simulink model "PV_MPPT"  (R2024a)
settings: Solver=ode23tb  StartTime=0.0  StopTime=10  RelTol=1e-4
libraries: spsSeriesRLCBranchLib x13, spsIGBTDiodeLib x6, spsGroundLib x3, spsSawtoothGeneratorLib x3, spsCurrentMeasurementLib x3, spsThreePhaseVIMeasurementLib x2, spsMeanLib x2, spsVoltageMeasurementLib x2, spspowerguiLib x1, simulink x1, spsDiodeLib x1, spsIGBTLib x1
settings Model: Creator=91889  LastModifiedBy=91889

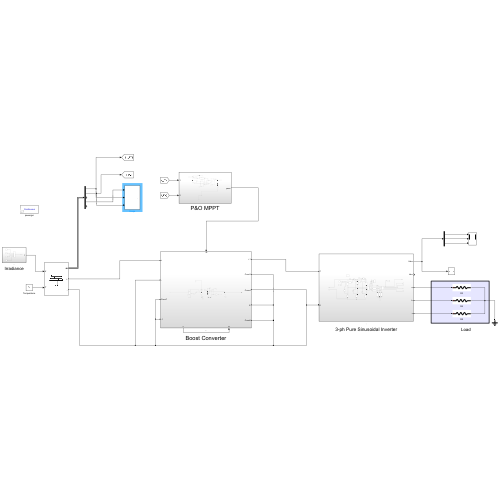
[thumbnail: Simulink's stored preview of the top-level diagram]
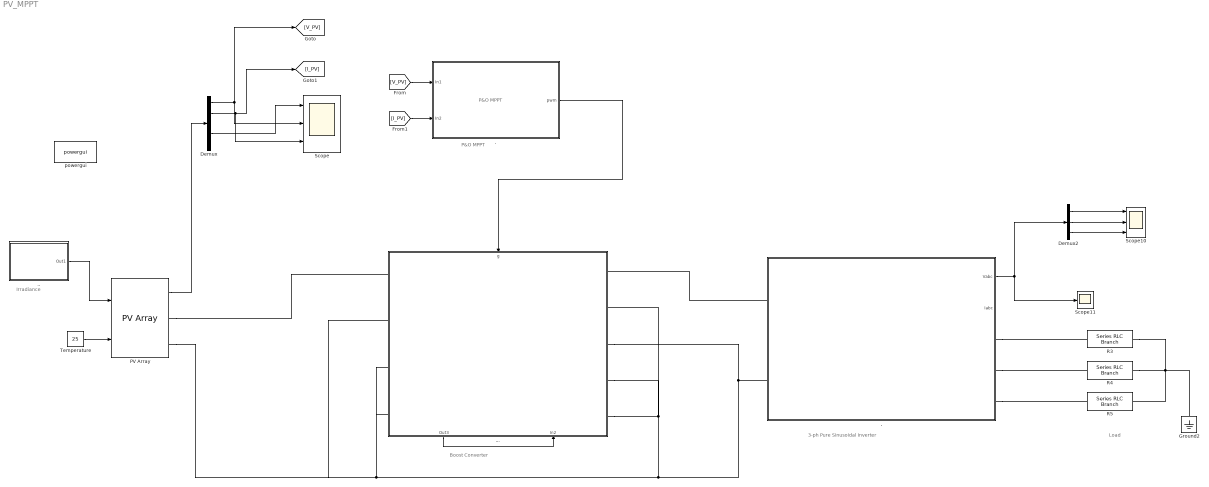
== system PV_MPPT ==
  note: Load
  note: 3-ph Pure Sinusoidal Inverter
  note: Boost Converter
  note: Irradiance
  note: P&O MPPT
  note: P&O MPPT
  , : Subsystem
  . : Subsystem
  .. : Subsystem
  ... : Subsystem
      settings: PortSchema="{\"entries\":[{\"content\":{\"sides\":[{\"content\":{\"connectorIds\":[\"LConn1\",\"LConn2\",\"LConn3\",\"LConn4\"]},\"type\":\"ConnectorPlacement.EquallySpacedRectSide\",\"uuid\":\"853841bf-2c6c-476b-8930-0dad7cd27bd4\"},{\"content\":{\"connectorIds\":[\"RConn1\",\"RConn2\",\"RConn3\",\"RConn4\",\"RConn5\"],\"side\":\"RIGHT\"},\"type\":\"ConnectorPlacement.EquallySpacedRectSide\",\"uuid\":\"d1ca2537-bf77-4a41-a82f-700dc7148288\"},{\"content\":{\"connectorIds\":[\"In1\"],\"side\":\"TOP\"},\"type\":\"ConnectorPlacement.EquallySpacedRectSide\",\"uuid\":\"50e3e9f4-8721-4df0-9f81-d71172613d0c\"},{\"content\":{\"connectorIds\":[\"Out1\",\"In2\"],\"side\":\"BOTTOM\"},\"type\":\"ConnectorPlacement.EquallySpacedRectSide\",\"uuid\":\"0662db4a-a60b-41ea-b11c-bd3a3f86f72a\"}]},\"type\":\"ConnectorPlacement.EquallySpacedConnector\",\"uuid\":\"eb88438f-1bf4-4f6a-82c1-55dd1ddf17b5\"}],\"packageUris\":[\"http://schema.mathworks.com/mf0/Connector/R2020b\"],\"version\":\"1.0\"}"
  Demux : Demux  Outputs=5
  Demux2 : Demux  Outputs=3
  Ground2 : spsGroundLib/Ground  LConnTagsString=a
  PV Array : spsPVArrayLib/PV Array  Npar=3  Nser=20  PlotType=array @ 1000 W/m2 & specified temperatures  S_vec="[ 1000  500  100 ]"  Temp_C_vec="[ 45 25  ]"  ModuleName=User-defined  PlotWhenSelected=off  Pm=213.15  Ncell=60  Voc=35  Isc=7.84  Vm=29  Im=7.35  beta_Voc_pc=-0.36099  alpha_Isc_pc=0.102  beta_Voc=-0.12635  alpha_Isc=0.0079968  IL=7.8812  I0=2.9282e-10  nI=0.94636  Rsh=184.8932  Rs=0.22133  RobustModel=off  RobustCellTemperature=313.3991  BAL=on  Tc=1e-6  Tfilter=5e-5
  R3 : spsSeriesRLCBranchLib/Series RLC Branch  LConnTagsString=__new0  RConnTagsString=__new0  BranchType=R  Resistance=10  Inductance=1e-3  SetiL0=off  InitialCurrent=0  Capacitance=1e-6  Setx0=off  InitialVoltage=0  Measurements=None
  R4 : spsSeriesRLCBranchLib/Series RLC Branch  LConnTagsString=__new0  RConnTagsString=__new0  BranchType=R  Resistance=10  Inductance=1e-3  SetiL0=off  InitialCurrent=0  Capacitance=1e-6  Setx0=off  InitialVoltage=0  Measurements=None
  R5 : spsSeriesRLCBranchLib/Series RLC Branch  LConnTagsString=__new0  RConnTagsString=__new0  BranchType=R  Resistance=10  Inductance=1e-3  SetiL0=off  InitialCurrent=0  Capacitance=1e-6  Setx0=off  InitialVoltage=0  Measurements=None
  Scope : Scope  NumInputPorts=3
  Scope10 : Scope  NumInputPorts=3
  Scope11 : Scope
  Temperature : Constant  Value=25
  powergui : sps_lib/powergui  Priority=1  SimulationMode=Continuous  SampleTime=50e-6  frequency=60  Iterations=50  frequencyindice=0  Pbase=100e6  ErrMax=1e-4  UnitsV=kV  UnitsW=MW  buscounter=0  FunctionMessages=off  echomessages=off  EnableUseOfTLC=off  CurrentSourceSwitches=off  DisableSnubberDevices=off  DisableRonSwitches=off  DisableVfSwitches=off  DisplayEquations=off  AutomaticDiscreteSolvers=off  SolverType=Tustin/Backward Euler (TBE)  Interpol=off  ExternalGateDelay=off  methode=off  Ts=100  x0status=blocks  SPID=on  SwTol=0  HookPort=off  NonlinearTolerance=1e-4  nMaxIteration=100  ContinueOnMaxIteration=off  RestoreLinks=warning  ResistiveCurrentMeasurement=off  Frange=[0:2:500]  Ylog=off  Xlog=on  ShowGrid=off  save=off  variable=ZData  structure=0  ZoomFFT=off  StartTime=0.0  cycles=1  DisplayStyle=1  fundamental=60  FreqAxis=off  MaxFrequency=1000  frequencyindicesteady=1  RmsSteady=1  display=off
  wires:
  Temperature/1 -> PV Array/2
  PV Array/1 -> Demux/1
  Demux/1 -> [V_PV], Scope/2
  Demux/2 -> Scope/3, [I_PV]
  Demux2/3 -> Scope10/3
  Demux2/1 -> Scope10/1
  ,/1(Vabc) -> Demux2/1, Scope11/1
  Demux2/2 -> Scope10/2
  ../1(Out1) -> PV Array/1
  [V_PV] -> ./1(In1)
  [I_PV] -> ./2(In2)
  ./1(pwm) -> .../1(g)
  .../1(Out3) -> .../2(In2)
  Demux/4 -> Scope/1
  connections:
  R3/RConn1 -- R5/RConn1 -- Ground2/LConn1 -- R4/RConn1
  ,/RConn1 -- R3/LConn1
  ,/RConn2 -- R4/LConn1
  ,/RConn3 -- R5/LConn1
  ,/LConn2 -- .../LConn2 -- PV Array/RConn2 -- .../LConn4 -- .../LConn3 -- .../RConn5 -- .../RConn4 -- .../RConn2 -- .../RConn3
  PV Array/RConn1 -- .../LConn1
  ,/LConn1 -- .../RConn1

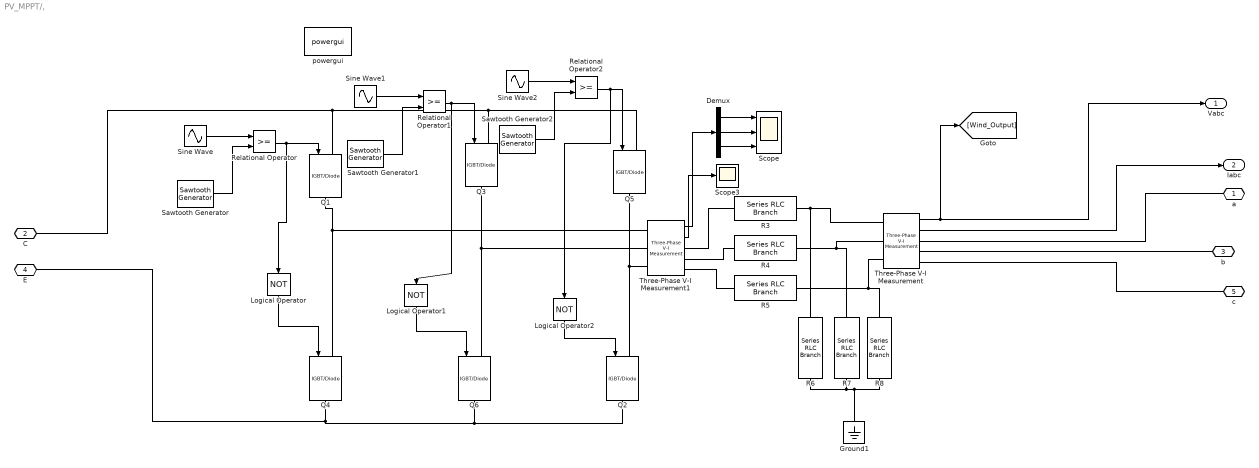
== system PV_MPPT/, ==
  Demux : Demux  Outputs=3
  Ground1 : spsGroundLib/Ground  LConnTagsString=a
  Logical Operator : Logic  Operator=NOT  AllPortsSameDT=off  OutDataTypeStr=boolean
  Logical Operator1 : Logic  Operator=NOT  AllPortsSameDT=off  OutDataTypeStr=boolean
  Logical Operator2 : Logic  Operator=NOT  AllPortsSameDT=off  OutDataTypeStr=boolean
  Q{1..6} (6 alike) : spsIGBTDiodeLib/IGBT//Diode  Ron=1e-3  Rs=1e5  Cs=inf  Measurements=off
  R3 : spsSeriesRLCBranchLib/Series RLC Branch  LConnTagsString=__new0  RConnTagsString=__new0  BranchType=L  Resistance=10  Inductance=80e-3  SetiL0=off  InitialCurrent=0  Capacitance=1e-6  Setx0=off  InitialVoltage=0  Measurements=None
  R4 : spsSeriesRLCBranchLib/Series RLC Branch  LConnTagsString=__new0  RConnTagsString=__new0  BranchType=L  Resistance=10  Inductance=80e-3  SetiL0=off  InitialCurrent=0  Capacitance=1e-6  Setx0=off  InitialVoltage=0  Measurements=None
  R5 : spsSeriesRLCBranchLib/Series RLC Branch  LConnTagsString=__new0  RConnTagsString=__new0  BranchType=L  Resistance=10  Inductance=80e-3  SetiL0=off  InitialCurrent=0  Capacitance=1e-6  Setx0=off  InitialVoltage=0  Measurements=None
  R6 : spsSeriesRLCBranchLib/Series RLC Branch  LConnTagsString=__new0  RConnTagsString=__new0  BranchType=C  Resistance=10  Inductance=80e-3  SetiL0=off  InitialCurrent=0  Capacitance=300e-6  Setx0=off  InitialVoltage=0  Measurements=None
  R7 : spsSeriesRLCBranchLib/Series RLC Branch  LConnTagsString=__new0  RConnTagsString=__new0  BranchType=C  Resistance=10  Inductance=80e-3  SetiL0=off  InitialCurrent=0  Capacitance=300e-6  Setx0=off  InitialVoltage=0  Measurements=None
  R8 : spsSeriesRLCBranchLib/Series RLC Branch  LConnTagsString=__new0  RConnTagsString=__new0  BranchType=C  Resistance=10  Inductance=80e-3  SetiL0=off  InitialCurrent=0  Capacitance=300e-6  Setx0=off  InitialVoltage=0  Measurements=None
  Relational Operator : RelationalOperator  OutDataTypeStr=boolean  InputSameDT=off
  Relational Operator1 : RelationalOperator  OutDataTypeStr=boolean  InputSameDT=off
  Relational Operator2 : RelationalOperator  OutDataTypeStr=boolean  InputSameDT=off
  Sawtooth Generator : spsSawtoothGeneratorLib/Sawtooth Generator  Freq=1000  Phase=180  Ts=0
  Sawtooth Generator1 : spsSawtoothGeneratorLib/Sawtooth Generator  Freq=1000  Phase=180  Ts=0
  Sawtooth Generator2 : spsSawtoothGeneratorLib/Sawtooth Generator  Freq=1000  Phase=180  Ts=0
  Scope : Scope  NumInputPorts=3
  Scope3 : Scope
  Sine Wave : Sin  Amplitude=0.9  Frequency=2*pi*50  SampleTime=0
  Sine Wave1 : Sin  Amplitude=0.9  Frequency=2*pi*50  Phase=120*(pi/180)  SampleTime=0
  Sine Wave2 : Sin  Amplitude=0.9  Frequency=2*pi*50  Phase=240*(pi/180)  SampleTime=0
  Three-Phase V-I Measurement : spsThreePhaseVIMeasurementLib/Three-Phase V-I Measurement  VoltageMeasurement=phase-to-phase  SetLabelV=off  LabelV=Vabc  Vpu=off  VpuLL=off  CurrentMeasurement=yes  SetLabelI=off  LabelI=Iabc  Ipu=off  Pbase=100e6  Vbase=500e3  OutputType=Complex  PhasorSimulation=off  PSBequivalent=0
  Three-Phase V-I Measurement1 : spsThreePhaseVIMeasurementLib/Three-Phase V-I Measurement  VoltageMeasurement=phase-to-phase  SetLabelV=off  LabelV=Vabc  Vpu=off  VpuLL=off  CurrentMeasurement=yes  SetLabelI=off  LabelI=Iabc  Ipu=off  Pbase=100e6  Vbase=500e3  OutputType=Complex  PhasorSimulation=off  PSBequivalent=0
  powergui : spspowerguiLib/powergui  Priority=1  SimulationMode=Continuous  SampleTime=50e-6  frequency=60  Iterations=50  frequencyindice=0  Pbase=100e6  ErrMax=1e-4  UnitsV=kV  UnitsW=MW  buscounter=0  FunctionMessages=off  echomessages=off  EnableUseOfTLC=off  CurrentSourceSwitches=off  DisableSnubberDevices=off  DisableRonSwitches=off  DisableVfSwitches=off  DisplayEquations=off  AutomaticDiscreteSolvers=off  SolverType=Tustin/Backward Euler (TBE)  Interpol=off  ExternalGateDelay=off  methode=off  Ts=100  x0status=blocks  SPID=off  SwTol=0  HookPort=off  NonlinearTolerance=1e-4  nMaxIteration=100  ContinueOnMaxIteration=off  RestoreLinks=warning  ResistiveCurrentMeasurement=off  Frange=[0:2:500]  Ylog=off  Xlog=on  ShowGrid=off  save=off  variable=ZData  structure=Vo  ZoomFFT=off  StartTime=0.0  cycles=1  DisplayStyle=1  fundamental=50  FreqAxis=on  MaxFrequency=1000  frequencyindicesteady=1  RmsSteady=1  display=off
  a : PMIOPort  Side=Right
  C : PMIOPort  Port=2  Side=Left
  b : PMIOPort  Port=3  Side=Right
  E : PMIOPort  Port=4  Side=Left
  c : PMIOPort  Port=5  Side=Right
  Vabc : Outport
  Iabc : Outport  Port=2
  wires:
  Relational Operator1/1 -> Q3/1, Logical Operator1/1
  Logical Operator/1 -> Q4/1
  Three-Phase V-I Measurement/1 -> [Wind_Output], Vabc/1
  Three-Phase V-I Measurement1/2 -> Scope3/1
  Logical Operator1/1 -> Q6/1
  Sawtooth Generator2/1 -> Relational Operator2/2
  Relational Operator2/1 -> Logical Operator2/1, Q5/1
  Logical Operator2/1 -> Q2/1
  Sawtooth Generator/1 -> Relational Operator/2
  Demux/1 -> Scope/1
  Three-Phase V-I Measurement1/1 -> Demux/1
  Relational Operator/1 -> Logical Operator/1, Q1/1
  Sawtooth Generator1/1 -> Relational Operator1/2
  Sine Wave/1 -> Relational Operator/1
  Three-Phase V-I Measurement/2 -> Iabc/1
  Sine Wave1/1 -> Relational Operator1/1
  Sine Wave2/1 -> Relational Operator2/1
  Demux/3 -> Scope/3
  Demux/2 -> Scope/2
  connections:
  R4/LConn1 -- Three-Phase V-I Measurement1/RConn2
  Q4/RConn1 -- Q6/RConn1 -- Q2/RConn1 -- E/RConn1
  Q5/LConn1 -- Q3/LConn1 -- Q1/LConn1 -- C/RConn1
  R6/LConn1 -- Three-Phase V-I Measurement/LConn1 -- R3/RConn1
  Three-Phase V-I Measurement1/LConn3 -- Q5/RConn1 -- Q2/LConn1
  Three-Phase V-I Measurement1/LConn2 -- Q3/RConn1 -- Q6/LConn1
  R7/LConn1 -- R4/RConn1 -- Three-Phase V-I Measurement/LConn2
  R5/LConn1 -- Three-Phase V-I Measurement1/RConn3
  Ground1/LConn1 -- R8/RConn1 -- R6/RConn1 -- R7/RConn1
  R8/LConn1 -- R5/RConn1 -- Three-Phase V-I Measurement/LConn3
  Three-Phase V-I Measurement/RConn3 -- c/RConn1
  Three-Phase V-I Measurement1/LConn1 -- Q1/RConn1 -- Q4/LConn1
  R3/LConn1 -- Three-Phase V-I Measurement1/RConn1
  Three-Phase V-I Measurement/RConn1 -- a/RConn1
  Three-Phase V-I Measurement/RConn2 -- b/RConn1

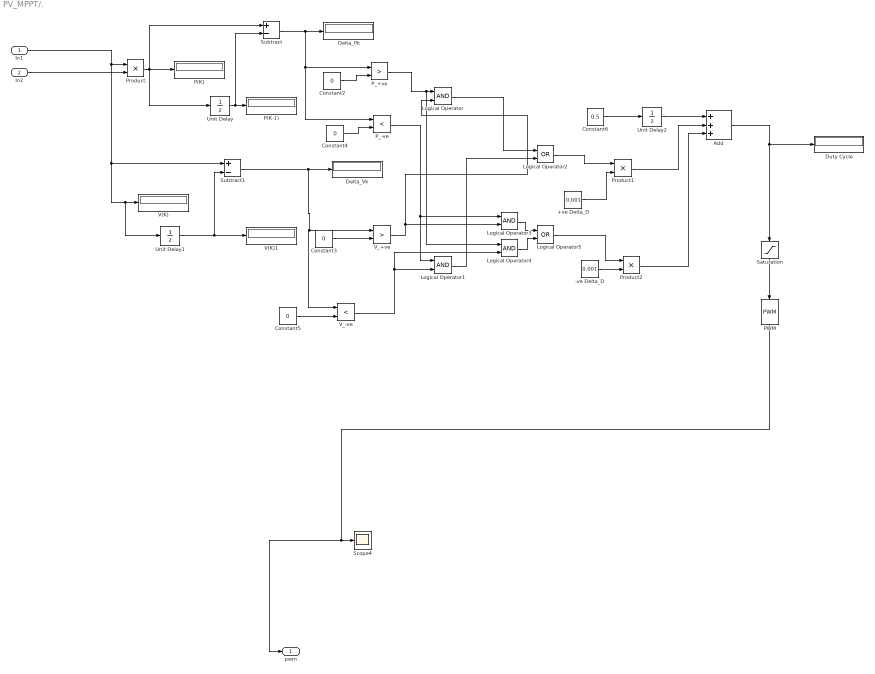
== system PV_MPPT/. ==
  In1 : Inport
  In2 : Inport  Port=2
  +ve Delta_D : Constant  Value=0.001
  -ve Delta_D : Constant  Value=0.001
  Add : Sum  Inputs=+++
  Constant{2..5} (4 alike) : Constant  Value=0
  Constant6 : Constant  Value=0.5
  Delta_Pk : Display
  Delta_Vk : Display
  Duty Cycle : Display
  Logical Operator{,1,3..4} (4 alike) : Logic  AllPortsSameDT=off  OutDataTypeStr=boolean
  Logical Operator2 : Logic  Operator=OR  AllPortsSameDT=off  OutDataTypeStr=boolean
  Logical Operator5 : Logic  Operator=OR  AllPortsSameDT=off  OutDataTypeStr=boolean
  P(K) : Display
  P(K-1) : Display
  PWM : simulink/Discontinuities/PWM  DisableCoverage=on  Period=50e-6  InitialDelay=0  DisallowZeroDutyCycle=off  RunAtFixedTimeIntervals=off  SampleTime=0.1
  P_+ve : RelationalOperator  Operator=>  OutDataTypeStr=boolean  RndMeth=Simplest  InputSameDT=off
  P_-ve : RelationalOperator  Operator=<  OutDataTypeStr=boolean  RndMeth=Simplest  InputSameDT=off
  Product : Product
  Product1 : Product
  Product2 : Product
  Saturation : Saturate  UpperLimit=0.9  LowerLimit=0.1
  Scope4 : Scope
  Subtract : Sum  Inputs=+-
  Subtract1 : Sum  Inputs=+-
  Unit Delay : UnitDelay  SampleTime=-1  HasFrameUpgradeWarning=on
  Unit Delay1 : UnitDelay  SampleTime=-1  HasFrameUpgradeWarning=on
  Unit Delay2 : UnitDelay  SampleTime=-1  HasFrameUpgradeWarning=on
  V(K) : Display
  V(K)1 : Display
  V_+ve : RelationalOperator  Operator=>  OutDataTypeStr=boolean  RndMeth=Simplest  InputSameDT=off
  V_-ve : RelationalOperator  Operator=<  OutDataTypeStr=boolean  RndMeth=Simplest  InputSameDT=off
  pwm : Outport
  wires:
  Product2/1 -> Add/3
  -ve Delta_D/1 -> Product2/2
  Product/1 -> Unit Delay/1, Subtract/1, P(K)/1
  In1/1 -> Subtract1/1, V(K)/1, Unit Delay1/1, Product/1
  +ve Delta_D/1 -> Product1/2
  V_+ve/1 -> Logical Operator/2, Logical Operator3/2
  Saturation/1 -> PWM/1
  Unit Delay1/1 -> Subtract1/2, V(K)1/1
  V_-ve/1 -> Logical Operator4/2, Logical Operator1/2
  Subtract1/1 -> V_-ve/1, V_+ve/1, Delta_Vk/1
  Logical Operator/1 -> Logical Operator2/1
  Logical Operator1/1 -> Logical Operator2/2
  Logical Operator4/1 -> Logical Operator5/2
  Add/1 -> Saturation/1, Duty Cycle/1
  Constant3/1 -> V_+ve/2
  P_+ve/1 -> Logical Operator4/1, Logical Operator/1
  Logical Operator3/1 -> Logical Operator5/1
  Constant5/1 -> V_-ve/2
  Unit Delay/1 -> Subtract/2, P(K-1)/1
  Unit Delay2/1 -> Add/1
  Subtract/1 -> Delta_Pk/1, P_-ve/1, P_+ve/1
  Constant4/1 -> P_-ve/2
  PWM/1 -> pwm/1, Scope4/1
  Constant6/1 -> Unit Delay2/1
  Product1/1 -> Add/2
  Logical Operator2/1 -> Product1/1
  Constant2/1 -> P_+ve/2
  P_-ve/1 -> Logical Operator3/1, Logical Operator1/1
  Logical Operator5/1 -> Product2/1
  In2/1 -> Product/2

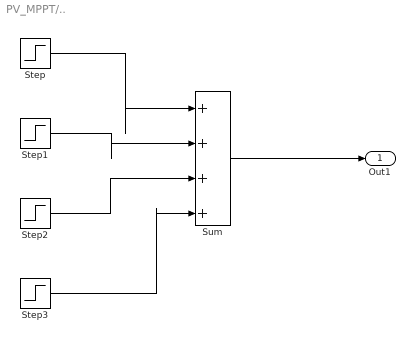
== system PV_MPPT/.. ==
  Step : Step  Time=0  Before=1200  After=1200  SampleTime=0
  Step1 : Step  Time=3  After=-300  SampleTime=0
  Step2 : Step  Time=5  After=-250  SampleTime=0
  Step3 : Step  Time=8  After=350  SampleTime=0
  Sum : Sum  Inputs=|++++
  Out1 : Outport
  wires:
  Step1/1 -> Sum/2
  Step/1 -> Sum/1
  Sum/1 -> Out1/1
  Step2/1 -> Sum/3
  Step3/1 -> Sum/4

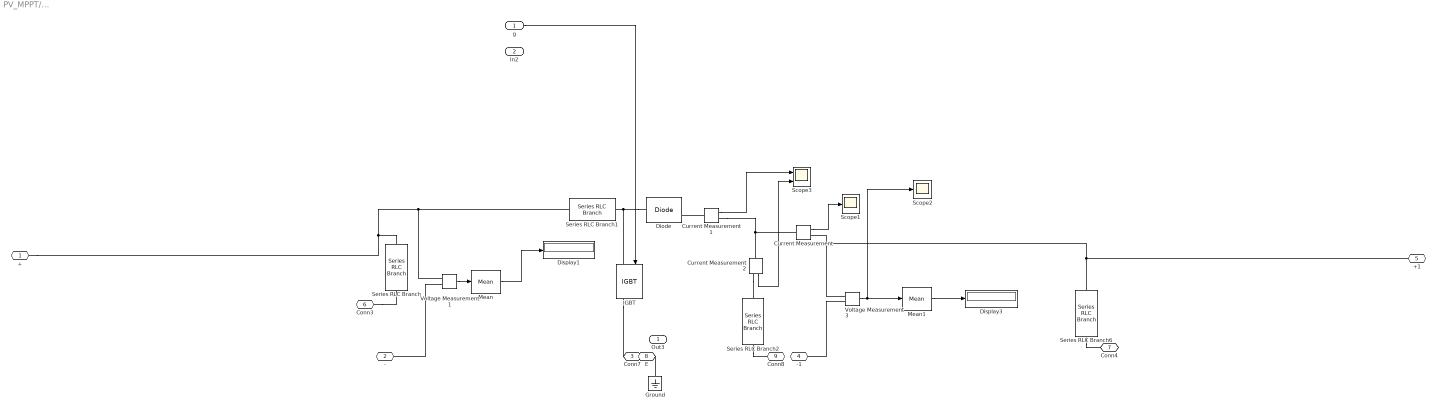
== system PV_MPPT/... ==
  g : Inport
  In2 : Inport  Port=2
  Current Measurement : spsCurrentMeasurementLib/Current Measurement  PhasorSimulation=off  OutputType=Complex  PSBequivalent=0
  Current Measurement1 : spsCurrentMeasurementLib/Current Measurement  PhasorSimulation=off  OutputType=Complex  PSBequivalent=0
  Current Measurement2 : spsCurrentMeasurementLib/Current Measurement  PhasorSimulation=off  OutputType=Complex  PSBequivalent=0
  Diode : spsDiodeLib/Diode  Ron=0.001  Lon=0  Vf=0.8  IC=0  UseSnubber=0  Rs=500  Cs=250e-9  Measurements=on
  Display1 : Display
  Display3 : Display
  Ground : spsGroundLib/Ground  LConnTagsString=a
  IGBT : spsIGBTLib/IGBT  Ron=0.001  Lon=0  Vf=1  Tf=1e-6  Tt=2e-6  IC=0  Rs=1e5  Cs=inf  Measurements=on
  Mean : spsMeanLib/Mean  Freq=60  Vinit=0  Ts=0
  Mean1 : spsMeanLib/Mean  Freq=60  Vinit=0  Ts=0
  Scope1 : Scope
  Scope2 : Scope
  Scope3 : Scope  NumInputPorts=2
  Series RLC Branch : spsSeriesRLCBranchLib/Series RLC Branch  LConnTagsString=__new0  RConnTagsString=__new0  BranchType=R  Resistance=100  Inductance=1e-3  SetiL0=off  InitialCurrent=0  Capacitance=1e-6  Setx0=off  InitialVoltage=0  Measurements=None
  Series RLC Branch1 : spsSeriesRLCBranchLib/Series RLC Branch  LConnTagsString=__new0  RConnTagsString=__new0  BranchType=L  Resistance=1  Inductance=5e-3  SetiL0=off  InitialCurrent=0  Capacitance=1e-6  Setx0=off  InitialVoltage=0  Measurements=None
  Series RLC Branch2 : spsSeriesRLCBranchLib/Series RLC Branch  LConnTagsString=__new0  RConnTagsString=__new0  BranchType=C  Resistance=1  Inductance=1e-3  SetiL0=off  InitialCurrent=0  Capacitance=1000e-6  Setx0=off  InitialVoltage=0  Measurements=None
  Series RLC Branch6 : spsSeriesRLCBranchLib/Series RLC Branch  LConnTagsString=__new0  RConnTagsString=__new0  BranchType=R  Resistance=10  Inductance=1e-3  SetiL0=off  InitialCurrent=0  Capacitance=32e-6  Setx0=off  InitialVoltage=0  Measurements=None
  Voltage Measurement1 : spsVoltageMeasurementLib/Voltage Measurement  PhasorSimulation=off  OutputType=Complex  PSBequivalent=0
  Voltage Measurement3 : spsVoltageMeasurementLib/Voltage Measurement  PhasorSimulation=off  OutputType=Complex  PSBequivalent=0
  + : PMIOPort  Side=Left
  - : PMIOPort  Port=2  Side=Left
  Conn7 : PMIOPort  Port=3  Side=Left
  -1 : PMIOPort  Port=4  Side=Left
  +1 : PMIOPort  Port=5  Side=Right
  Conn3 : PMIOPort  Port=6  Side=Right
  Conn4 : PMIOPort  Port=7  Side=Right
  E : PMIOPort  Port=8  Side=Right
  Conn8 : PMIOPort  Port=9  Side=Right
  Out3 : Outport
  wires:
  Mean/1 -> Display1/1
  Voltage Measurement1/1 -> Mean/1
  Mean1/1 -> Display3/1
  Current Measurement/1 -> Scope1/1
  g/1 -> IGBT/1
  Current Measurement2/1 -> Scope3/2
  Voltage Measurement3/1 -> Mean1/1, Scope2/1
  Current Measurement1/1 -> Scope3/1
  connections:
  Voltage Measurement1/LConn1 -- Series RLC Branch1/LConn1 -- +/RConn1 -- Series RLC Branch/LConn1
  Diode/LConn1 -- Series RLC Branch1/RConn1 -- IGBT/LConn1
  Series RLC Branch6/RConn1 -- Conn4/RConn1
  Current Measurement2/RConn1 -- Series RLC Branch2/LConn1
  Current Measurement1/RConn1 -- Current Measurement/LConn1 -- Current Measurement2/LConn1
  Current Measurement1/LConn1 -- Diode/RConn1
  IGBT/RConn1 -- E/RConn1
  Current Measurement/RConn1 -- +1/RConn1 -- Series RLC Branch6/LConn1 -- Voltage Measurement3/LConn1
  Series RLC Branch2/RConn1 -- Conn8/RConn1
  Conn3/RConn1 -- Series RLC Branch/RConn1
  Ground/LConn1 -- Conn7/RConn1
  Voltage Measurement3/LConn2 -- -1/RConn1
  Voltage Measurement1/LConn2 -- -/RConn1
